simulink model "CONTROL_PLANTA"  (R2018b)
settings: Solver=ode45  StartTime=0.0  StopTime=15  RelTol=1e-3
values from neighbouring files (symbols this model uses):
  Kc = Kc-h*Kc    (= 5.939406)    [ALGORITMO_FINAL.m]    (also in Optimizacion.m = Kc+h*Kc)
  Kc2 = Kc    (= 5.939406)    [ALGORITMO_FINAL.m]    (also in Optimizacion.m = Kc)
  td = td-h*td    (= 0.2351014875)    [ALGORITMO_FINAL.m]    (also in Optimizacion.m = td+h*td)
  ti = ti-h*ti    (= 0.94040595)    [ALGORITMO_FINAL.m]    (also in Optimizacion.m = ti+h*ti)
  ti2 = ti    (= 0.94040595)    [ALGORITMO_FINAL.m]    (also in Optimizacion.m = ti)
undefined symbols (not defined in the file or in its folder): den1, den2, den3, num1, num2, num3
libraries: simulink x2
settings Model: Creator=Sergio  LastModifiedBy=DELL
settings OptimizationCC: LifeSpan=inf
settings DebuggingCC: SFExecutionAtInitializationDiag=none
settings HardwareCC: ProdBitPerSizeT=32  ProdBitPerPtrDiffT=32  ProdWordSize=32  ProdHWDeviceType=Specified
settings SFSimCC: SimUseLocalCustomCode=off
settings RTWCC: RTWUseLocalCustomCode=off
settings CodeAppCC: StateflowObjectComments=on

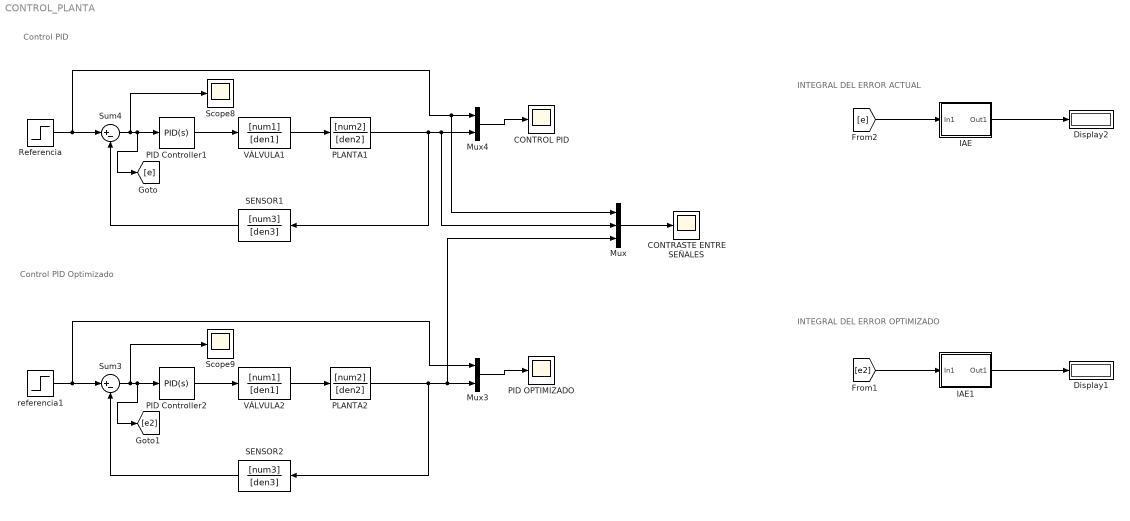
== system CONTROL_PLANTA ==
  note: Control PID
  note: Control PID Optimizado
  note: INTEGRAL DEL ERROR ACTUAL
  note: INTEGRAL DEL ERROR OPTIMIZADO
  CONTRASTE ENTRE SEÑALES : Scope
  CONTROL PID : Scope
  Display1 : Display
  Display2 : Display
  IAE : Subsystem
  IAE1 : Subsystem
  Mux : Mux  Inputs=3
  Mux3 : Mux  Inputs=2
  Mux4 : Mux  Inputs=2
  PID Controller1 : simulink/Continuous/PID Controller  Controller=PID  Form=Parallel  TimeDomain=Continuous-time  SampleTime=-1  IntegratorMethod=Forward Euler  FilterMethod=Forward Euler  ControllerParametersSource=internal  P=Kc  I=Kc*(1/ti)  D=Kc*td  UseFilter=on  N=100  TunerSelectOption=Transfer Function Based (PID Tuner App)  InitialConditionSource=internal  InitialConditionForIntegrator=0  InitialConditionForFilter=0  DifferentiatorICPrevScaledInput=0  ExternalReset=none  TrackingMode=off  Kt=1  LimitOutput=off  UpperSaturationLimit=inf  LowerSaturationLimit=-inf  LinearizeAsGain=on  AntiWindupMode=none  Kb=1  POutMin=[]  POutMax=[]  IOutMin=[]  IOutMax=[]  DOutMin=[]  DOutMax=[]  NOutMin=[]  NOutMax=[]  SumOutMin=[]  SumOutMax=[]  SaturationOutMin=[]  SaturationOutMax=[]  PParamMin=[]  PParamMax=[]  IParamMin=[]  IParamMax=[]  DParamMin=[]  DParamMax=[]  NParamMin=[]  NParamMax=[]  KbParamMin=[]  KbParamMax=[]  KtParamMin=[]  KtParamMax=[]  KbOutMin=[]  KbOutMax=[]  KtOutMin=[]  KtOutMax=[]  IntegratorOutMin=[]  IntegratorOutMax=[]  FilterOutMin=[]  FilterOutMax=[]  SumI1OutMin=[]  SumI1OutMax=[]  SumI2OutMin=[]  SumI2OutMax=[]  SumI3OutMin=[]  SumI3OutMax=[]  SumI4OutMin=[]  SumI4OutMax=[]  SumDOutMin=[]  SumDOutMax=[]  DifferentiatorOutMin=[]  DifferentiatorOutMax=[]  FilterDiffOutCoefMin=[]  FilterDiffOutCoefMax=[]  ReciprocalOutMin=[]  ReciprocalOutMax=[]  SumDenOutMin=[]  SumDenOutMax=[]  SumNumOutMin=[]  SumNumOutMax=[]  DivideOutMin=[]  DivideOutMax=[]  IntegratorContinuousStateAttributes=''  IntegratorStateMustResolveToSignalObject=off  IntegratorRTWStateStorageClass=Auto  FilterContinuousStateAttributes=''  FilterStateMustResolveToSignalObject=off  FilterRTWStateStorageClass=Auto  ParallelPVariant=InternalParameters  IdealPVariant=Disabled  IVariant=InternalParameters  DVariant=InternalParameters  IntegratorVariant=Continuous  SatVariant=Disabled  AWVariant=Passthrough  PCopyVariant=Disabled  TRVariant=Disabled  FdbkBlocksVariant=Forward  IdealPFdbkVariant=Disabled  SatFdbkVariant=Disabled  DerivativeFilterVariant=ContFilter  NVariant=InternalParameters  NCopyVariant=Disabled  FilterICVariant=InternalICsFilter  IntegratorICVariant=InternalICs  ExternalResetVariant=Disabled  TRSumVariant=Passthrough  SumFdbkVariant=Disabled  SumVariant=Sum_PID
  PID Controller2 : simulink/Continuous/PID Controller  Controller=PID  Form=Parallel  TimeDomain=Continuous-time  SampleTime=-1  IntegratorMethod=Forward Euler  FilterMethod=Forward Euler  ControllerParametersSource=internal  P=Kc2  I=Kc2*(1/ti2)  D=Kc2*td  UseFilter=on  N=100  TunerSelectOption=Transfer Function Based (PID Tuner App)  InitialConditionSource=internal  InitialConditionForIntegrator=0  InitialConditionForFilter=0  DifferentiatorICPrevScaledInput=0  ExternalReset=none  TrackingMode=off  Kt=1  LimitOutput=off  UpperSaturationLimit=inf  LowerSaturationLimit=-inf  LinearizeAsGain=on  AntiWindupMode=none  Kb=1  POutMin=[]  POutMax=[]  IOutMin=[]  IOutMax=[]  DOutMin=[]  DOutMax=[]  NOutMin=[]  NOutMax=[]  SumOutMin=[]  SumOutMax=[]  SaturationOutMin=[]  SaturationOutMax=[]  PParamMin=[]  PParamMax=[]  IParamMin=[]  IParamMax=[]  DParamMin=[]  DParamMax=[]  NParamMin=[]  NParamMax=[]  KbParamMin=[]  KbParamMax=[]  KtParamMin=[]  KtParamMax=[]  KbOutMin=[]  KbOutMax=[]  KtOutMin=[]  KtOutMax=[]  IntegratorOutMin=[]  IntegratorOutMax=[]  FilterOutMin=[]  FilterOutMax=[]  SumI1OutMin=[]  SumI1OutMax=[]  SumI2OutMin=[]  SumI2OutMax=[]  SumI3OutMin=[]  SumI3OutMax=[]  SumI4OutMin=[]  SumI4OutMax=[]  SumDOutMin=[]  SumDOutMax=[]  DifferentiatorOutMin=[]  DifferentiatorOutMax=[]  FilterDiffOutCoefMin=[]  FilterDiffOutCoefMax=[]  ReciprocalOutMin=[]  ReciprocalOutMax=[]  SumDenOutMin=[]  SumDenOutMax=[]  SumNumOutMin=[]  SumNumOutMax=[]  DivideOutMin=[]  DivideOutMax=[]  IntegratorContinuousStateAttributes=''  IntegratorStateMustResolveToSignalObject=off  IntegratorRTWStateStorageClass=Auto  FilterContinuousStateAttributes=''  FilterStateMustResolveToSignalObject=off  FilterRTWStateStorageClass=Auto  ParallelPVariant=InternalParameters  IdealPVariant=Disabled  IVariant=InternalParameters  DVariant=InternalParameters  IntegratorVariant=Continuous  SatVariant=Disabled  AWVariant=Passthrough  PCopyVariant=Disabled  TRVariant=Disabled  FdbkBlocksVariant=Forward  IdealPFdbkVariant=Disabled  SatFdbkVariant=Disabled  DerivativeFilterVariant=ContFilter  NVariant=InternalParameters  NCopyVariant=Disabled  FilterICVariant=InternalICsFilter  IntegratorICVariant=InternalICs  ExternalResetVariant=Disabled  TRSumVariant=Passthrough  SumFdbkVariant=Disabled  SumVariant=Sum_PID
  PID OPTIMIZADO : Scope
  PLANTA1 : TransferFcn  Numerator=[num2]  Denominator=[den2]
  PLANTA2 : TransferFcn  Numerator=[num2]  Denominator=[den2]
  Referencia : Step  SampleTime=0
  SENSOR1 : TransferFcn  Numerator=[num3]  Denominator=[den3]
  SENSOR2 : TransferFcn  Numerator=[num3]  Denominator=[den3]
  Scope8 : Scope
  Scope9 : Scope
  Sum3 : Sum  Inputs=|+-
  Sum4 : Sum  Inputs=|+-
  VÁLVULA1 : TransferFcn  Numerator=[num1]  Denominator=[den1]
  VÁLVULA2 : TransferFcn  Numerator=[num1]  Denominator=[den1]
  referencia1 : Step  SampleTime=0
  wires:
  Referencia/1 -> Mux/1, Mux4/1, Sum4/1
  PLANTA1/1 -> SENSOR1/1, Mux/2, Mux4/2
  Mux4/1 -> CONTROL PID/1
  Sum4/1 -> Scope8/1, [e], PID Controller1/1
  PID Controller1/1 -> VÁLVULA1/1
  VÁLVULA1/1 -> PLANTA1/1
  SENSOR1/1 -> Sum4/2
  IAE/1(Out1) -> Display2/1
  [e] -> IAE/1(In1)
  VÁLVULA2/1 -> PLANTA2/1
  PLANTA2/1 -> SENSOR2/1, Mux/3, Mux3/2
  referencia1/1 -> Mux3/1, Sum3/1
  Mux3/1 -> PID OPTIMIZADO/1
  SENSOR2/1 -> Sum3/2
  PID Controller2/1 -> VÁLVULA2/1
  Sum3/1 -> Scope9/1, [e2], PID Controller2/1
  IAE1/1(Out1) -> Display1/1
  [e2] -> IAE1/1(In1)
  Mux/1 -> CONTRASTE ENTRE SEÑALES/1

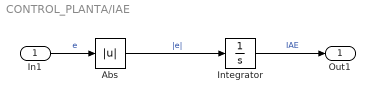
== system CONTROL_PLANTA/IAE ==
  In1 : Inport
  Abs : Abs
  Integrator : Integrator
  Out1 : Outport
  wires:
  Integrator/1 -> Out1/1  "IAE"
  In1/1 -> Abs/1  "e"
  Abs/1 -> Integrator/1  "|e|"

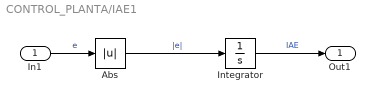
== system CONTROL_PLANTA/IAE1 ==
  In1 : Inport
  Abs : Abs
  Integrator : Integrator
  Out1 : Outport
  wires:
  Integrator/1 -> Out1/1  "IAE"
  In1/1 -> Abs/1  "e"
  Abs/1 -> Integrator/1  "|e|"
